simulink model "simCreateKinematicsNL_feedbackLinearizationCtrl"  (Simulink 7.9)
settings: Solver=ode3  StartTime=0.0  StopTime=1.43  FixedStep=0.0001  RelTol=1e-3
libraries: simulink x1
settings Model: Creator=Jon  LastModifiedBy=jon
settings DataIOCC: SaveState=on
settings DebuggingCC: FcnCallInpInsideContextMsg=Use local settings  StrictBusMsg=Warning
settings GRTTargetCC: CombineOutputUpdateFcns=off  GRTInterface=on

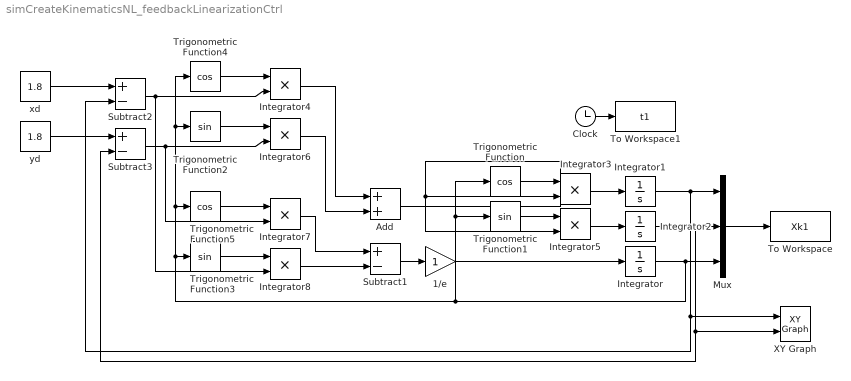
== system simCreateKinematicsNL_feedbackLinearizationCtrl ==
  1/e : Gain
  Add : Sum
  Clock : Clock
  Integrator : Integrator  InitialCondition=0.3925
  Integrator1 : Integrator  InitialCondition=0.15
  Integrator2 : Integrator  InitialCondition=0.15
  Integrator{3..8} (6 alike) : Product  RndMeth=Zero
  Mux : Mux  Inputs=3
  Subtract1 : Sum  Inputs=+-
  Subtract2 : Sum  Inputs=+-
  Subtract3 : Sum  Inputs=+-
  To Workspace : ToWorkspace  VariableName=Xk1  SampleTime=-1
  To Workspace1 : ToWorkspace  VariableName=t1  SampleTime=-1
  Trigonometric Function : Trigonometry  Operator=cos
  Trigonometric Function1 : Trigonometry
  Trigonometric Function2 : Trigonometry
  Trigonometric Function3 : Trigonometry
  Trigonometric Function4 : Trigonometry  Operator=cos
  Trigonometric Function5 : Trigonometry  Operator=cos
  XY Graph : simulink/Sinks/XY Graph  xmin=0  xmax=2  ymin=0  ymax=2  st=-1
  xd : Constant  Value=1.8
  yd : Constant  Value=1.8
  wires:
  Trigonometric Function/1 -> Integrator3/1
  Add/1 -> Integrator3/2, Integrator5/2
  Trigonometric Function1/1 -> Integrator5/1
  Integrator3/1 -> Integrator1/1
  Integrator5/1 -> Integrator2/1
  Integrator/1 -> Mux/3, Trigonometric Function1/1, Trigonometric Function/1, Trigonometric Function4/1, Trigonometric Function2/1, Trigonometric Function5/1, Trigonometric Function3/1
  Subtract1/1 -> 1/e/1
  Integrator1/1 -> Mux/1, Subtract2/2, XY Graph/1
  Integrator2/1 -> Mux/2, Subtract3/2, XY Graph/2
  Mux/1 -> To Workspace/1
  Clock/1 -> To Workspace1/1
  xd/1 -> Subtract2/1
  yd/1 -> Subtract3/1
  Trigonometric Function4/1 -> Integrator4/1
  Trigonometric Function2/1 -> Integrator6/1
  Subtract2/1 -> Integrator4/2, Integrator8/2
  Subtract3/1 -> Integrator6/2, Integrator7/2
  Integrator4/1 -> Add/1
  Integrator6/1 -> Add/2
  1/e/1 -> Integrator/1
  Trigonometric Function3/1 -> Integrator8/1
  Trigonometric Function5/1 -> Integrator7/1
  Integrator8/1 -> Subtract1/2
  Integrator7/1 -> Subtract1/1
